simulink model "ft33_project2"  (R2024a)
settings: Solver=VariableStepAuto  StartTime=0.0  StopTime=10.0  RelTol=1e-3
undefined symbols (not defined in the file or in its folder): ft33_project2_copy, Subsystem16, xc7z020clg484
libraries: hdlBasic x111, vmcUtilities x1
(part 1 of 2)
settings Model: Creator=ft33  LastModifiedBy=ft33

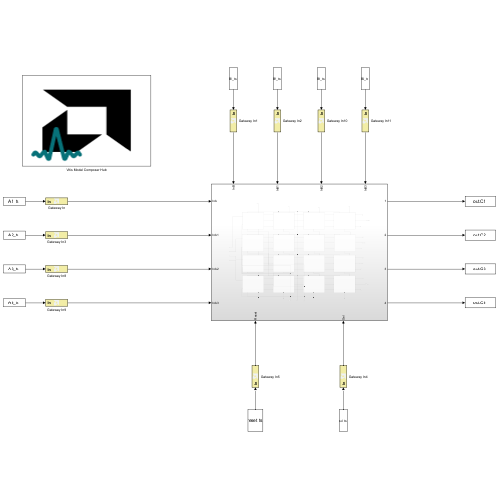
[thumbnail: Simulink's stored preview of the top-level diagram]
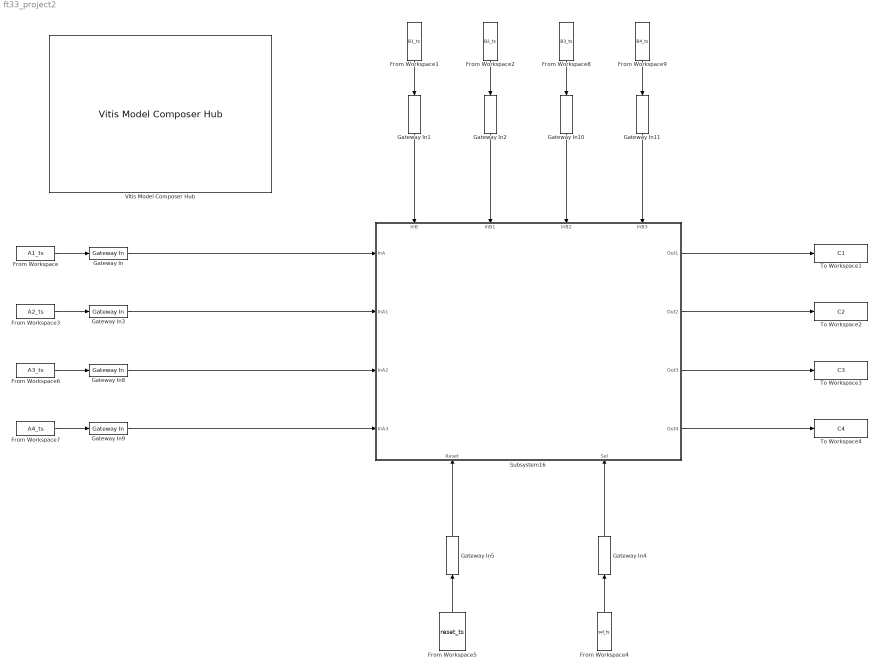
== system ft33_project2 ==
  From Workspace : FromWorkspace  VariableName=A1_ts
  From Workspace1 : FromWorkspace  VariableName=B1_ts
  From Workspace2 : FromWorkspace  VariableName=B2_ts
  From Workspace3 : FromWorkspace  VariableName=A2_ts
  From Workspace4 : FromWorkspace  VariableName=sel_ts
  From Workspace5 : FromWorkspace  VariableName=reset_ts
  From Workspace6 : FromWorkspace  VariableName=A3_ts
  From Workspace7 : FromWorkspace  VariableName=A4_ts
  From Workspace8 : FromWorkspace  VariableName=B3_ts
  From Workspace9 : FromWorkspace  VariableName=B4_ts
  Gateway In{,1..3,8..11} (8 alike) : hdlBasic/Gateway In  gui_display_data_type=Fixed-point  arith_type=Signed (2's comp)  n_bits=16  bin_pt=0  preci_type=Single  exp_width=8  frac_width=24  rows=1  columns=1  quantization="Round  (unbiased: +/- Inf)"  overflow=Saturate  period=1  UseAsADC=off  ADCChannel='1'  interface=None  automatic_assignment=on  address_offset=hex2dec('00')  intf_name=''  intf_description=''  default_value=0  timing_constraint=None  locs_specified=off  LOCs={}  io_standard={}  inherit_from_input=off  hdl_port=on  XmcBlockStatus=1  maskContainerNames=group4  block_type=gatewayin  block_config=sysgen:gateway_in_config  block_width_w=590  block_height_w=620  block_width=640  block_height=850
  Gateway In4 : hdlBasic/Gateway In  gui_display_data_type=Boolean  arith_type=Boolean  n_bits=16  bin_pt=14  preci_type=Single  exp_width=8  frac_width=24  rows=1  columns=1  quantization="Round  (unbiased: +/- Inf)"  overflow=Saturate  period=1  UseAsADC=off  ADCChannel='1'  interface=None  automatic_assignment=on  address_offset=hex2dec('00')  intf_name=''  intf_description=''  default_value=0  timing_constraint=None  locs_specified=off  LOCs={}  io_standard={}  inherit_from_input=off  hdl_port=on  XmcBlockStatus=1  maskContainerNames=group4  block_type=gatewayin  block_config=sysgen:gateway_in_config  block_width_w=590  block_height_w=620  block_width=640  block_height=850
  Gateway In5 : hdlBasic/Gateway In  gui_display_data_type=Boolean  arith_type=Boolean  n_bits=16  bin_pt=14  preci_type=Single  exp_width=8  frac_width=24  rows=1  columns=1  quantization="Round  (unbiased: +/- Inf)"  overflow=Saturate  period=1  UseAsADC=off  ADCChannel='1'  interface=None  automatic_assignment=on  address_offset=hex2dec('00')  intf_name=''  intf_description=''  default_value=0  timing_constraint=None  locs_specified=off  LOCs={}  io_standard={}  inherit_from_input=off  hdl_port=on  XmcBlockStatus=1  maskContainerNames=group4  block_type=gatewayin  block_config=sysgen:gateway_in_config  block_width_w=590  block_height_w=620  block_width=640  block_height=850
  Subsystem16 : Subsystem
      settings: PortSchema="{\"entries\":[{\"content\":{\"sides\":[{\"content\":{\"connectorIds\":[\"In1\",\"In2\",\"In3\",\"In4\"]},\"type\":\"ConnectorPlacement.EquallySpacedRectSide\",\"uuid\":\"57fd51eb-b579-40c5-a499-8811be9ed02c\"},{\"content\":{\"connectorIds\":[\"Out1\",\"Out2\",\"Out3\",\"Out4\"],\"side\":\"RIGHT\"},\"type\":\"ConnectorPlacement.EquallySpacedRectSide\",\"uuid\":\"f81d02a0-f624-4ba0-87e4-de8c38e96c8a\"},{\"content\":{\"connectorIds\":[\"In5\",\"In6\",\"In7\",\"In8\"],\"side\":\"TOP\"},\"type\":\"ConnectorPlacement.EquallySpacedRectSide\",\"uuid\":\"b728b957-3fa5-4fc3-9d0e-7e74a65ebaf5\"},{\"content\":{\"connectorIds\":[\"In9\",\"In10\"],\"side\":\"BOTTOM\"},\"type\":\"ConnectorPlacement.EquallySpacedRectSide\",\"uuid\":\"48c0373e-0401-44d8-8aa7-85e5a3af1fce\"}]},\"type\":\"ConnectorPlacement.EquallySpacedConnector\",\"uuid\":\"375c5da9-2b8b-40e9-8e99-56d50ddf0ba4\"}],\"packageUris\":[\"http://schema.mathworks.com/mf0/Connector/R2020b\"],\"version\":\"1.0\"}"
  To Workspace1 : ToWorkspace  VariableName=C1  SampleTime=-1
  To Workspace2 : ToWorkspace  VariableName=C2  SampleTime=-1
  To Workspace3 : ToWorkspace  VariableName=C3  SampleTime=-1
  To Workspace4 : ToWorkspace  VariableName=C4  SampleTime=-1
  Vitis Model Composer Hub : vmcUtilities/Vitis Model Composer Hub  Tag=genX  CodeGeneration=off  SubsystemName=Subsystem16  BlockHierPath=ft33_project2_copy/Subsystem16  CompilationType=HDLCompilation  SubsystemType=HDLNode  ExportTypeV2=IP Catalog  StartColumn=1  NumberOfColumns=1  TargetDirectory=C:/ELEC522/ft33/Project2_Copy/ResourceAnalysis  exportDesign=off  analyzeDesign=on  validateDesignOnHw=off  ExportType=AI Engines  IpVendor=xilinx.com  IpLibrary=hls  IpVersion=1.0  IpHWLanguage=Verilog  AieCompilerOptions={}  AieSimulatorOptions={}  CreateTestbench=on  TestbenchStackSize=10  RunRtlSim=off  RunCSim=off  RunAieSim=off  AieSimTimeout=50000  RunAieSimProfiling=off  LaunchVitisAnalyzer=off  PlotOutput=off  RunX86Sim=off  X86SimTimeout=10  GenHwImage=off  GenLibadfXo=off  GenHwValidationCode=off  PlatformType=Not Specified  HwSystemType=Baremetal  HwValidationTarget=hw  ProjDevice=ZedBoard Zynq Evaluation and Development Kit (xc7z020clg484-1)  ProjDevicePart=xc7z020clg484-1  AIEType=None  SamplePeriod=-1  ClockFrequency=200  DataPathParallelism=1  xilinxfamily=zynq  part=xc7z020  speed=-1  package=clg484  directory=C:/ELEC522/ft33/Project2_Copy/ResourceAnalysis\ip\Subsystem16\src  testbench=on  incr_netlist=off  synthesis_tool=Vivado  clock_wrapper=Clock Enables  dbl_ovrd=According to Block Masks  dcm_input_clock_period=10  sysclk_period=10  simulink_period=1  eval_field=0  IPInfoJsonString="{\"DUTSubsystemName\":\"Subsystem16\",\"HDLSubsystem\":{\"SubsystemName\":\"Subsystem16\",\"IPName\":\"Subsystem16\",\"IPLibrary\":\"VMC\",\"IPVendor\":\"User Company\",\"IPVersion\":\"1.0\",\"TargetDirectory\":\"C:/ELEC522/ft33/Project2_Copy/ResourceAnalysis\",\"SubsystemDir\":\"C:/ELEC522/ft33/Project2_Copy/ResourceAnalysis\\\\ip\\\\Subsystem16\",\"FreqHz\":\"100000000\"},\"SubsystemTag\":\"HDLNode\"}"  LogFileName=C:\ELEC522\ft33\Project2_Copy\ResourceAnalysis\model_composer.log  NThreads=4  IPConfigFile=C:\Users\ft33\AppData\Local\Temp\vmctmp-8900646231309001291\ft33_project2_copy_ipconfig.json
  wires:
  From Workspace/1 -> Gateway In/1
  From Workspace1/1 -> Gateway In1/1
  From Workspace2/1 -> Gateway In2/1
  From Workspace4/1 -> Gateway In4/1
  From Workspace5/1 -> Gateway In5/1
  From Workspace6/1 -> Gateway In8/1
  From Workspace7/1 -> Gateway In9/1
  From Workspace8/1 -> Gateway In10/1
  From Workspace9/1 -> Gateway In11/1
  From Workspace3/1 -> Gateway In3/1
  Gateway In1/1 -> Subsystem16/5(InB)
  Gateway In2/1 -> Subsystem16/6(InB1)
  Gateway In10/1 -> Subsystem16/7(InB2)
  Gateway In11/1 -> Subsystem16/8(InB3)
  Gateway In/1 -> Subsystem16/1(InA)
  Gateway In3/1 -> Subsystem16/2(InA1)
  Gateway In8/1 -> Subsystem16/3(InA2)
  Gateway In9/1 -> Subsystem16/4(InA3)
  Gateway In4/1 -> Subsystem16/10(Sel)
  Gateway In5/1 -> Subsystem16/9(Reset)
  Subsystem16/1(Out1) -> To Workspace1/1
  Subsystem16/2(Out2) -> To Workspace2/1
  Subsystem16/3(Out3) -> To Workspace3/1
  Subsystem16/4(Out4) -> To Workspace4/1

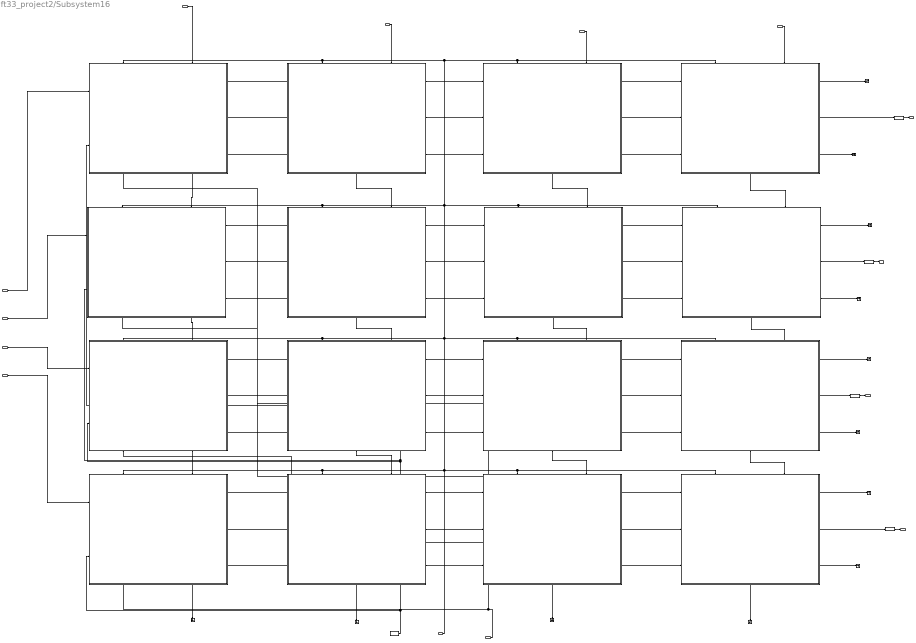
== system ft33_project2/Subsystem16 ==
  InA : Inport
  InA1 : Inport  Port=2
  InA2 : Inport  Port=3
  InA3 : Inport  Port=4
  InB : Inport  Port=5
  InB1 : Inport  Port=6
  InB2 : Inport  Port=7
  InB3 : Inport  Port=8
  Reset : Inport  Port=9
  Sel : Inport  Port=10
  Constant : hdlBasic/Constant  const=0  gui_display_data_type=Fixed-point  arith_type=Unsigned  n_bits=16  bin_pt=0  preci_type=Single  exp_width=8  frac_width=24  explicit_period=off  period=1  XmcBlockStatus=1  maskContainerNames=tabcontainer1  block_type=constant  block_config=sysgen:Constant_config
  Gateway Out{1..4} (4 alike) : hdlBasic/Gateway Out  inherit_from_input=off  bool_to_boolean=off  hdl_port=on  rows=1  columns=1  UseAsDAC=off  DACChannel='1'  interface=None  automatic_assignment=on  address_offset=hex2dec('00')  intf_name=''  intf_description=''  timing_constraint=None  locs_specified=off  LOCs={}  io_standard={}  XmcBlockStatus=1  maskContainerNames=group4  block_type=gatewayout  block_config=sysgen:gateway_out_config  block_width_w=590  block_height_w=620  block_width=620  block_height=750
  Subsystem : Subsystem
      settings: PortSchema="{\"entries\":[{\"content\":{\"sides\":[{\"content\":{\"connectorIds\":[\"In1\",\"In2\"]},\"type\":\"ConnectorPlacement.EquallySpacedRectSide\",\"uuid\":\"273aa0e1-58eb-4403-bf5b-6776102820e6\"},{\"content\":{\"connectorIds\":[\"Out1\",\"Out2\",\"Out3\"],\"side\":\"RIGHT\"},\"type\":\"ConnectorPlacement.EquallySpacedRectSide\",\"uuid\":\"5c33fd88-0c62-4daf-a6d0-9a1459fa340e\"},{\"content\":{\"connectorIds\":[\"In3\",\"In4\"],\"side\":\"TOP\"},\"type\":\"ConnectorPlacement.EquallySpacedRectSide\",\"uuid\":\"2690377b-a45b-49c1-9b26-3eb080cd9126\"},{\"content\":{\"connectorIds\":[\"In5\",\"Out4\"],\"side\":\"BOTTOM\"},\"type\":\"ConnectorPlacement.EquallySpacedRectSide\",\"uuid\":\"fadedb7c-b790-413e-aa9f-7f3073b39ea6\"}]},\"type\":\"ConnectorPlacement.EquallySpacedConnector\",\"uuid\":\"6510aed3-e923-4205-a634-903eef17da44\"}],\"packageUris\":[\"http://schema.mathworks.com/mf0/Connector/R2020b\"],\"version\":\"1.0\"}"
  Subsystem1 : Subsystem
      settings: PortSchema="{\"entries\":[{\"content\":{\"sides\":[{\"content\":{\"connectorIds\":[\"In1\",\"In2\",\"In3\"]},\"type\":\"ConnectorPlacement.EquallySpacedRectSide\",\"uuid\":\"273aa0e1-58eb-4403-bf5b-6776102820e6\"},{\"content\":{\"connectorIds\":[\"Out1\",\"Out2\",\"Out3\"],\"side\":\"RIGHT\"},\"type\":\"ConnectorPlacement.EquallySpacedRectSide\",\"uuid\":\"5c33fd88-0c62-4daf-a6d0-9a1459fa340e\"},{\"content\":{\"connectorIds\":[\"In4\",\"In5\"],\"side\":\"TOP\"},\"type\":\"ConnectorPlacement.EquallySpacedRectSide\",\"uuid\":\"2690377b-a45b-49c1-9b26-3eb080cd9126\"},{\"content\":{\"connectorIds\":[\"Out4\"],\"side\":\"BOTTOM\"},\"type\":\"ConnectorPlacement.EquallySpacedRectSide\",\"uuid\":\"fadedb7c-b790-413e-aa9f-7f3073b39ea6\"}]},\"type\":\"ConnectorPlacement.EquallySpacedConnector\",\"uuid\":\"6510aed3-e923-4205-a634-903eef17da44\"}],\"packageUris\":[\"http://schema.mathworks.com/mf0/Connector/R2020b\"],\"version\":\"1.0\"}"
  Subsystem10 : Subsystem
      settings: PortSchema="{\"entries\":[{\"content\":{\"sides\":[{\"content\":{\"connectorIds\":[\"In1\",\"In2\",\"In3\"]},\"type\":\"ConnectorPlacement.EquallySpacedRectSide\",\"uuid\":\"273aa0e1-58eb-4403-bf5b-6776102820e6\"},{\"content\":{\"connectorIds\":[\"Out1\",\"Out2\",\"Out3\"],\"side\":\"RIGHT\"},\"type\":\"ConnectorPlacement.EquallySpacedRectSide\",\"uuid\":\"5c33fd88-0c62-4daf-a6d0-9a1459fa340e\"},{\"content\":{\"connectorIds\":[\"In4\",\"In5\"],\"side\":\"TOP\"},\"type\":\"ConnectorPlacement.EquallySpacedRectSide\",\"uuid\":\"2690377b-a45b-49c1-9b26-3eb080cd9126\"},{\"content\":{\"connectorIds\":[\"Out4\"],\"side\":\"BOTTOM\"},\"type\":\"ConnectorPlacement.EquallySpacedRectSide\",\"uuid\":\"fadedb7c-b790-413e-aa9f-7f3073b39ea6\"}]},\"type\":\"ConnectorPlacement.EquallySpacedConnector\",\"uuid\":\"6510aed3-e923-4205-a634-903eef17da44\"}],\"packageUris\":[\"http://schema.mathworks.com/mf0/Connector/R2020b\"],\"version\":\"1.0\"}"
  Subsystem11 : Subsystem
      settings: PortSchema="{\"entries\":[{\"content\":{\"sides\":[{\"content\":{\"connectorIds\":[\"In1\",\"In2\",\"In3\"]},\"type\":\"ConnectorPlacement.EquallySpacedRectSide\",\"uuid\":\"273aa0e1-58eb-4403-bf5b-6776102820e6\"},{\"content\":{\"connectorIds\":[\"Out1\",\"Out2\",\"Out3\"],\"side\":\"RIGHT\"},\"type\":\"ConnectorPlacement.EquallySpacedRectSide\",\"uuid\":\"5c33fd88-0c62-4daf-a6d0-9a1459fa340e\"},{\"content\":{\"connectorIds\":[\"In4\",\"In5\"],\"side\":\"TOP\"},\"type\":\"ConnectorPlacement.EquallySpacedRectSide\",\"uuid\":\"2690377b-a45b-49c1-9b26-3eb080cd9126\"},{\"content\":{\"connectorIds\":[\"Out4\"],\"side\":\"BOTTOM\"},\"type\":\"ConnectorPlacement.EquallySpacedRectSide\",\"uuid\":\"fadedb7c-b790-413e-aa9f-7f3073b39ea6\"}]},\"type\":\"ConnectorPlacement.EquallySpacedConnector\",\"uuid\":\"6510aed3-e923-4205-a634-903eef17da44\"}],\"packageUris\":[\"http://schema.mathworks.com/mf0/Connector/R2020b\"],\"version\":\"1.0\"}"
  Subsystem12 : Subsystem
      settings: PortSchema="{\"entries\":[{\"content\":{\"sides\":[{\"content\":{\"connectorIds\":[\"In1\",\"In2\",\"In3\"]},\"type\":\"ConnectorPlacement.EquallySpacedRectSide\",\"uuid\":\"273aa0e1-58eb-4403-bf5b-6776102820e6\"},{\"content\":{\"connectorIds\":[\"Out1\",\"Out2\",\"Out3\"],\"side\":\"RIGHT\"},\"type\":\"ConnectorPlacement.EquallySpacedRectSide\",\"uuid\":\"5c33fd88-0c62-4daf-a6d0-9a1459fa340e\"},{\"content\":{\"connectorIds\":[\"In4\",\"In5\"],\"side\":\"TOP\"},\"type\":\"ConnectorPlacement.EquallySpacedRectSide\",\"uuid\":\"2690377b-a45b-49c1-9b26-3eb080cd9126\"},{\"content\":{\"connectorIds\":[\"Out4\"],\"side\":\"BOTTOM\"},\"type\":\"ConnectorPlacement.EquallySpacedRectSide\",\"uuid\":\"fadedb7c-b790-413e-aa9f-7f3073b39ea6\"}]},\"type\":\"ConnectorPlacement.EquallySpacedConnector\",\"uuid\":\"6510aed3-e923-4205-a634-903eef17da44\"}],\"packageUris\":[\"http://schema.mathworks.com/mf0/Connector/R2020b\"],\"version\":\"1.0\"}"
  Subsystem13 : Subsystem
      settings: PortSchema="{\"entries\":[{\"content\":{\"sides\":[{\"content\":{\"connectorIds\":[\"In1\",\"In2\",\"In3\"]},\"type\":\"ConnectorPlacement.EquallySpacedRectSide\",\"uuid\":\"273aa0e1-58eb-4403-bf5b-6776102820e6\"},{\"content\":{\"connectorIds\":[\"Out1\",\"Out2\",\"Out3\"],\"side\":\"RIGHT\"},\"type\":\"ConnectorPlacement.EquallySpacedRectSide\",\"uuid\":\"5c33fd88-0c62-4daf-a6d0-9a1459fa340e\"},{\"content\":{\"connectorIds\":[\"In4\",\"In5\"],\"side\":\"TOP\"},\"type\":\"ConnectorPlacement.EquallySpacedRectSide\",\"uuid\":\"2690377b-a45b-49c1-9b26-3eb080cd9126\"},{\"content\":{\"connectorIds\":[\"Out4\"],\"side\":\"BOTTOM\"},\"type\":\"ConnectorPlacement.EquallySpacedRectSide\",\"uuid\":\"fadedb7c-b790-413e-aa9f-7f3073b39ea6\"}]},\"type\":\"ConnectorPlacement.EquallySpacedConnector\",\"uuid\":\"6510aed3-e923-4205-a634-903eef17da44\"}],\"packageUris\":[\"http://schema.mathworks.com/mf0/Connector/R2020b\"],\"version\":\"1.0\"}"
  Subsystem14 : Subsystem
      settings: PortSchema="{\"entries\":[{\"content\":{\"sides\":[{\"content\":{\"connectorIds\":[\"In1\",\"In2\",\"In3\"]},\"type\":\"ConnectorPlacement.EquallySpacedRectSide\",\"uuid\":\"273aa0e1-58eb-4403-bf5b-6776102820e6\"},{\"content\":{\"connectorIds\":[\"Out1\",\"Out2\",\"Out3\"],\"side\":\"RIGHT\"},\"type\":\"ConnectorPlacement.EquallySpacedRectSide\",\"uuid\":\"5c33fd88-0c62-4daf-a6d0-9a1459fa340e\"},{\"content\":{\"connectorIds\":[\"In4\",\"In5\"],\"side\":\"TOP\"},\"type\":\"ConnectorPlacement.EquallySpacedRectSide\",\"uuid\":\"2690377b-a45b-49c1-9b26-3eb080cd9126\"},{\"content\":{\"connectorIds\":[\"Out4\"],\"side\":\"BOTTOM\"},\"type\":\"ConnectorPlacement.EquallySpacedRectSide\",\"uuid\":\"fadedb7c-b790-413e-aa9f-7f3073b39ea6\"}]},\"type\":\"ConnectorPlacement.EquallySpacedConnector\",\"uuid\":\"6510aed3-e923-4205-a634-903eef17da44\"}],\"packageUris\":[\"http://schema.mathworks.com/mf0/Connector/R2020b\"],\"version\":\"1.0\"}"
  Subsystem15 : Subsystem
      settings: PortSchema="{\"entries\":[{\"content\":{\"sides\":[{\"content\":{\"connectorIds\":[\"In1\",\"In2\",\"In3\"]},\"type\":\"ConnectorPlacement.EquallySpacedRectSide\",\"uuid\":\"273aa0e1-58eb-4403-bf5b-6776102820e6\"},{\"content\":{\"connectorIds\":[\"Out1\",\"Out2\",\"Out3\"],\"side\":\"RIGHT\"},\"type\":\"ConnectorPlacement.EquallySpacedRectSide\",\"uuid\":\"5c33fd88-0c62-4daf-a6d0-9a1459fa340e\"},{\"content\":{\"connectorIds\":[\"In4\",\"In5\"],\"side\":\"TOP\"},\"type\":\"ConnectorPlacement.EquallySpacedRectSide\",\"uuid\":\"2690377b-a45b-49c1-9b26-3eb080cd9126\"},{\"content\":{\"connectorIds\":[\"Out4\"],\"side\":\"BOTTOM\"},\"type\":\"ConnectorPlacement.EquallySpacedRectSide\",\"uuid\":\"fadedb7c-b790-413e-aa9f-7f3073b39ea6\"}]},\"type\":\"ConnectorPlacement.EquallySpacedConnector\",\"uuid\":\"6510aed3-e923-4205-a634-903eef17da44\"}],\"packageUris\":[\"http://schema.mathworks.com/mf0/Connector/R2020b\"],\"version\":\"1.0\"}"
  Subsystem2 : Subsystem
      settings: PortSchema="{\"entries\":[{\"content\":{\"sides\":[{\"content\":{\"connectorIds\":[\"In1\",\"In2\"]},\"type\":\"ConnectorPlacement.EquallySpacedRectSide\",\"uuid\":\"273aa0e1-58eb-4403-bf5b-6776102820e6\"},{\"content\":{\"connectorIds\":[\"Out1\",\"Out2\",\"Out3\"],\"side\":\"RIGHT\"},\"type\":\"ConnectorPlacement.EquallySpacedRectSide\",\"uuid\":\"5c33fd88-0c62-4daf-a6d0-9a1459fa340e\"},{\"content\":{\"connectorIds\":[\"In3\",\"In4\"],\"side\":\"TOP\"},\"type\":\"ConnectorPlacement.EquallySpacedRectSide\",\"uuid\":\"2690377b-a45b-49c1-9b26-3eb080cd9126\"},{\"content\":{\"connectorIds\":[\"In5\",\"Out4\"],\"side\":\"BOTTOM\"},\"type\":\"ConnectorPlacement.EquallySpacedRectSide\",\"uuid\":\"fadedb7c-b790-413e-aa9f-7f3073b39ea6\"}]},\"type\":\"ConnectorPlacement.EquallySpacedConnector\",\"uuid\":\"6510aed3-e923-4205-a634-903eef17da44\"}],\"packageUris\":[\"http://schema.mathworks.com/mf0/Connector/R2020b\"],\"version\":\"1.0\"}"
  Subsystem3 : Subsystem
      settings: PortSchema="{\"entries\":[{\"content\":{\"sides\":[{\"content\":{\"connectorIds\":[\"In1\",\"In2\",\"In3\"]},\"type\":\"ConnectorPlacement.EquallySpacedRectSide\",\"uuid\":\"273aa0e1-58eb-4403-bf5b-6776102820e6\"},{\"content\":{\"connectorIds\":[\"Out1\",\"Out2\",\"Out3\"],\"side\":\"RIGHT\"},\"type\":\"ConnectorPlacement.EquallySpacedRectSide\",\"uuid\":\"5c33fd88-0c62-4daf-a6d0-9a1459fa340e\"},{\"content\":{\"connectorIds\":[\"In4\",\"In5\"],\"side\":\"TOP\"},\"type\":\"ConnectorPlacement.EquallySpacedRectSide\",\"uuid\":\"2690377b-a45b-49c1-9b26-3eb080cd9126\"},{\"content\":{\"connectorIds\":[\"Out4\"],\"side\":\"BOTTOM\"},\"type\":\"ConnectorPlacement.EquallySpacedRectSide\",\"uuid\":\"fadedb7c-b790-413e-aa9f-7f3073b39ea6\"}]},\"type\":\"ConnectorPlacement.EquallySpacedConnector\",\"uuid\":\"6510aed3-e923-4205-a634-903eef17da44\"}],\"packageUris\":[\"http://schema.mathworks.com/mf0/Connector/R2020b\"],\"version\":\"1.0\"}"
  Subsystem4 : Subsystem
      settings: PortSchema="{\"entries\":[{\"content\":{\"sides\":[{\"content\":{\"connectorIds\":[\"In1\",\"In2\"]},\"type\":\"ConnectorPlacement.EquallySpacedRectSide\",\"uuid\":\"273aa0e1-58eb-4403-bf5b-6776102820e6\"},{\"content\":{\"connectorIds\":[\"Out1\",\"Out2\",\"Out3\"],\"side\":\"RIGHT\"},\"type\":\"ConnectorPlacement.EquallySpacedRectSide\",\"uuid\":\"5c33fd88-0c62-4daf-a6d0-9a1459fa340e\"},{\"content\":{\"connectorIds\":[\"In3\",\"In4\"],\"side\":\"TOP\"},\"type\":\"ConnectorPlacement.EquallySpacedRectSide\",\"uuid\":\"2690377b-a45b-49c1-9b26-3eb080cd9126\"},{\"content\":{\"connectorIds\":[\"In5\",\"Out4\"],\"side\":\"BOTTOM\"},\"type\":\"ConnectorPlacement.EquallySpacedRectSide\",\"uuid\":\"fadedb7c-b790-413e-aa9f-7f3073b39ea6\"}]},\"type\":\"ConnectorPlacement.EquallySpacedConnector\",\"uuid\":\"6510aed3-e923-4205-a634-903eef17da44\"}],\"packageUris\":[\"http://schema.mathworks.com/mf0/Connector/R2020b\"],\"version\":\"1.0\"}"
  Subsystem5 : Subsystem
      settings: PortSchema="{\"entries\":[{\"content\":{\"sides\":[{\"content\":{\"connectorIds\":[\"In1\",\"In2\"]},\"type\":\"ConnectorPlacement.EquallySpacedRectSide\",\"uuid\":\"273aa0e1-58eb-4403-bf5b-6776102820e6\"},{\"content\":{\"connectorIds\":[\"Out1\",\"Out2\",\"Out3\"],\"side\":\"RIGHT\"},\"type\":\"ConnectorPlacement.EquallySpacedRectSide\",\"uuid\":\"5c33fd88-0c62-4daf-a6d0-9a1459fa340e\"},{\"content\":{\"connectorIds\":[\"In3\",\"In4\"],\"side\":\"TOP\"},\"type\":\"ConnectorPlacement.EquallySpacedRectSide\",\"uuid\":\"2690377b-a45b-49c1-9b26-3eb080cd9126\"},{\"content\":{\"connectorIds\":[\"In5\",\"Out4\"],\"side\":\"BOTTOM\"},\"type\":\"ConnectorPlacement.EquallySpacedRectSide\",\"uuid\":\"fadedb7c-b790-413e-aa9f-7f3073b39ea6\"}]},\"type\":\"ConnectorPlacement.EquallySpacedConnector\",\"uuid\":\"6510aed3-e923-4205-a634-903eef17da44\"}],\"packageUris\":[\"http://schema.mathworks.com/mf0/Connector/R2020b\"],\"version\":\"1.0\"}"
  Subsystem6 : Subsystem
      settings: PortSchema="{\"entries\":[{\"content\":{\"sides\":[{\"content\":{\"connectorIds\":[\"In1\",\"In2\",\"In3\"]},\"type\":\"ConnectorPlacement.EquallySpacedRectSide\",\"uuid\":\"273aa0e1-58eb-4403-bf5b-6776102820e6\"},{\"content\":{\"connectorIds\":[\"Out1\",\"Out2\",\"Out3\"],\"side\":\"RIGHT\"},\"type\":\"ConnectorPlacement.EquallySpacedRectSide\",\"uuid\":\"5c33fd88-0c62-4daf-a6d0-9a1459fa340e\"},{\"content\":{\"connectorIds\":[\"In4\",\"In5\"],\"side\":\"TOP\"},\"type\":\"ConnectorPlacement.EquallySpacedRectSide\",\"uuid\":\"2690377b-a45b-49c1-9b26-3eb080cd9126\"},{\"content\":{\"connectorIds\":[\"Out4\"],\"side\":\"BOTTOM\"},\"type\":\"ConnectorPlacement.EquallySpacedRectSide\",\"uuid\":\"fadedb7c-b790-413e-aa9f-7f3073b39ea6\"}]},\"type\":\"ConnectorPlacement.EquallySpacedConnector\",\"uuid\":\"6510aed3-e923-4205-a634-903eef17da44\"}],\"packageUris\":[\"http://schema.mathworks.com/mf0/Connector/R2020b\"],\"version\":\"1.0\"}"
  Subsystem7 : Subsystem
      settings: PortSchema="{\"entries\":[{\"content\":{\"sides\":[{\"content\":{\"connectorIds\":[\"In1\",\"In2\",\"In3\"]},\"type\":\"ConnectorPlacement.EquallySpacedRectSide\",\"uuid\":\"273aa0e1-58eb-4403-bf5b-6776102820e6\"},{\"content\":{\"connectorIds\":[\"Out1\",\"Out2\",\"Out3\"],\"side\":\"RIGHT\"},\"type\":\"ConnectorPlacement.EquallySpacedRectSide\",\"uuid\":\"5c33fd88-0c62-4daf-a6d0-9a1459fa340e\"},{\"content\":{\"connectorIds\":[\"In4\",\"In5\"],\"side\":\"TOP\"},\"type\":\"ConnectorPlacement.EquallySpacedRectSide\",\"uuid\":\"2690377b-a45b-49c1-9b26-3eb080cd9126\"},{\"content\":{\"connectorIds\":[\"Out4\"],\"side\":\"BOTTOM\"},\"type\":\"ConnectorPlacement.EquallySpacedRectSide\",\"uuid\":\"fadedb7c-b790-413e-aa9f-7f3073b39ea6\"}]},\"type\":\"ConnectorPlacement.EquallySpacedConnector\",\"uuid\":\"6510aed3-e923-4205-a634-903eef17da44\"}],\"packageUris\":[\"http://schema.mathworks.com/mf0/Connector/R2020b\"],\"version\":\"1.0\"}"
  Subsystem8 : Subsystem
      settings: PortSchema="{\"entries\":[{\"content\":{\"sides\":[{\"content\":{\"connectorIds\":[\"In1\",\"In2\",\"In3\"]},\"type\":\"ConnectorPlacement.EquallySpacedRectSide\",\"uuid\":\"273aa0e1-58eb-4403-bf5b-6776102820e6\"},{\"content\":{\"connectorIds\":[\"Out1\",\"Out2\",\"Out3\"],\"side\":\"RIGHT\"},\"type\":\"ConnectorPlacement.EquallySpacedRectSide\",\"uuid\":\"5c33fd88-0c62-4daf-a6d0-9a1459fa340e\"},{\"content\":{\"connectorIds\":[\"In4\",\"In5\"],\"side\":\"TOP\"},\"type\":\"ConnectorPlacement.EquallySpacedRectSide\",\"uuid\":\"2690377b-a45b-49c1-9b26-3eb080cd9126\"},{\"content\":{\"connectorIds\":[\"Out4\"],\"side\":\"BOTTOM\"},\"type\":\"ConnectorPlacement.EquallySpacedRectSide\",\"uuid\":\"fadedb7c-b790-413e-aa9f-7f3073b39ea6\"}]},\"type\":\"ConnectorPlacement.EquallySpacedConnector\",\"uuid\":\"6510aed3-e923-4205-a634-903eef17da44\"}],\"packageUris\":[\"http://schema.mathworks.com/mf0/Connector/R2020b\"],\"version\":\"1.0\"}"
  Subsystem9 : Subsystem
      settings: PortSchema="{\"entries\":[{\"content\":{\"sides\":[{\"content\":{\"connectorIds\":[\"In1\",\"In2\",\"In3\"]},\"type\":\"ConnectorPlacement.EquallySpacedRectSide\",\"uuid\":\"273aa0e1-58eb-4403-bf5b-6776102820e6\"},{\"content\":{\"connectorIds\":[\"Out1\",\"Out2\",\"Out3\"],\"side\":\"RIGHT\"},\"type\":\"ConnectorPlacement.EquallySpacedRectSide\",\"uuid\":\"5c33fd88-0c62-4daf-a6d0-9a1459fa340e\"},{\"content\":{\"connectorIds\":[\"In4\",\"In5\"],\"side\":\"TOP\"},\"type\":\"ConnectorPlacement.EquallySpacedRectSide\",\"uuid\":\"2690377b-a45b-49c1-9b26-3eb080cd9126\"},{\"content\":{\"connectorIds\":[\"Out4\"],\"side\":\"BOTTOM\"},\"type\":\"ConnectorPlacement.EquallySpacedRectSide\",\"uuid\":\"fadedb7c-b790-413e-aa9f-7f3073b39ea6\"}]},\"type\":\"ConnectorPlacement.EquallySpacedConnector\",\"uuid\":\"6510aed3-e923-4205-a634-903eef17da44\"}],\"packageUris\":[\"http://schema.mathworks.com/mf0/Connector/R2020b\"],\"version\":\"1.0\"}"
  Terminator{,1..11} (12 alike) : Terminator
  Out1 : Outport
  Out2 : Outport  Port=2
  Out3 : Outport  Port=3
  Out4 : Outport  Port=4
  wires:
  Subsystem5/4(OutB) -> Terminator/1  "ShiftB"
  Reset/1 -> Subsystem5/5(Reset), Subsystem4/5(Reset), Subsystem2/5(Reset), Subsystem/5(ResetIn)
  Subsystem3/1(OutA) -> Subsystem15/1(InA)  "ShiftB"
  Constant/1 -> Subsystem5/2(ShiftIn), Subsystem4/2(ShiftIn), Subsystem2/2(ShiftIn), Subsystem/2(ShiftIn)
  InB2/1 -> Subsystem14/5(InB)
  Subsystem1/1(OutA) -> Subsystem14/1(InA)  "ShiftB"
  Subsystem12/4(OutB) -> Subsystem13/5(InB)  "ShiftB"
  Subsystem6/4(OutB) -> Subsystem7/5(InB)  "ShiftB"
  InB/1 -> Subsystem/4(InB)
  Subsystem13/2(ShiftOut) -> Gateway Out3/1
  Sel/1 -> Subsystem11/4(Select), Subsystem9/4(Select), Subsystem7/4(Select), Subsystem5/3(Select), Subsystem10/4(Select), Subsystem8/4(Select), Subsystem6/4(Select), Subsystem4/3(Select), Subsystem13/4(Select), Subsystem15/4(Select), Subsystem3/4(Select), Subsystem2/3(Select), Subsystem14/4(Select), Subsystem12/4(Select), Subsystem1/4(Select), Subsystem/3(Select)
  Subsystem15/2(ShiftOut) -> Subsystem13/2(ShiftIn)  "ShiftOutput"
  Subsystem13/1(OutA) -> Terminator6/1  "ShiftA"
  InA2/1 -> Subsystem4/1(InA)
  Subsystem11/1(OutA) -> Terminator4/1  "ShiftA"
  Subsystem10/1(OutA) -> Terminator5/1  "ShiftA"
  Subsystem11/4(OutB) -> Terminator3/1  "ShiftB"
  Subsystem14/1(OutA) -> Subsystem12/1(InA)  "ShiftA"
  Subsystem14/4(OutB) -> Subsystem15/5(InB)  "ShiftB"
  Subsystem15/1(OutA) -> Subsystem13/1(InA)  "ShiftA"
  Subsystem3/4(OutB) -> Subsystem6/5(InB)  "ShiftB"
  Subsystem10/2(ShiftOut) -> Gateway Out2/1
  Subsystem7/4(OutB) -> Terminator1/1  "ShiftB"
  Subsystem2/4(OutB) -> Subsystem4/4(InB)  "ShiftB"
  Gateway Out4/1 -> Out4/1
  Subsystem/4(OutB) -> Subsystem2/4(InB)  "ShiftB"
  Subsystem3/2(ShiftOut) -> Subsystem15/2(ShiftIn)  "ShiftA"
  Subsystem/2(ShiftOut) -> Subsystem1/2(ShiftIn)  "ShiftOutput"
  InA/1 -> Subsystem/1(InA)
  Subsystem12/1(OutA) -> Terminator7/1  "ShiftA"
  Subsystem2/2(ShiftOut) -> Subsystem3/2(ShiftIn)  "ShiftOutput"
  Subsystem4/4(OutB) -> Subsystem5/4(InB)  "ShiftB"
  Subsystem8/4(OutB) -> Subsystem9/5(InB)  "ShiftB"
  Subsystem15/4(OutB) -> Subsystem8/5(InB)  "ShiftB"
  Subsystem9/4(OutB) -> Terminator2/1  "ShiftB"
  Subsystem10/4(OutB) -> Subsystem11/5(InB)  "ShiftB"
  Subsystem13/4(OutB) -> Subsystem10/5(InB)  "ShiftB"
  Subsystem1/4(OutB) -> Subsystem3/5(InB)  "ShiftB"
  Subsystem2/1(OutA) -> Subsystem3/1(InA)  "ShiftA"
  InA3/1 -> Subsystem5/1(InA)
  Subsystem/1(OutA) -> Subsystem1/1(InA)  "ShiftA"
  Gateway Out2/1 -> Out3/1
  Gateway Out3/1 -> Out2/1
  Gateway Out1/1 -> Out1/1
  InA1/1 -> Subsystem2/1(InA)
  InB3/1 -> Subsystem12/5(InB)
  InB1/1 -> Subsystem1/5(InB)
  Subsystem1/2(ShiftOut) -> Subsystem14/2(ShiftIn)  "ShiftOutput"
  Subsystem14/2(ShiftOut) -> Subsystem12/2(ShiftIn)  "ShiftOutput"
  Subsystem12/2(ShiftOut) -> Gateway Out1/1  "ShiftOutput"
  Subsystem11/2(ShiftOut) -> Gateway Out4/1  "ShiftOutput"
  Subsystem/3(ResetOut) -> Subsystem1/3(ResetIn)
  Subsystem1/3(Out1) -> Subsystem14/3(ResetIn)
  Subsystem14/3(ResetOut) -> Subsystem12/3(ResetIn)
  Subsystem12/3(ResetOut) -> Terminator8/1
  Subsystem2/3(ResetOut) -> Subsystem3/3(ResetIn)
  Subsystem3/3(ResetOut) -> Subsystem15/3(ResetIn)
  Subsystem15/3(ResetOut) -> Subsystem13/3(ResetIn)
  Subsystem13/3(ResetOut) -> Terminator9/1
  Subsystem4/1(OutA) -> Subsystem6/1(InA)  "ShiftA"
  Subsystem4/2(ShiftOut) -> Subsystem6/2(ShiftIn)  "ShiftOutput"
  Subsystem4/3(ResetOut) -> Subsystem6/3(ResetIn)
  Subsystem6/3(ResetOut) -> Subsystem8/3(ResetIn)
  Subsystem6/2(ShiftOut) -> Subsystem8/2(ShiftIn)  "ShiftA"
  Subsystem6/1(OutA) -> Subsystem8/1(InA)  "ShiftB"
  Subsystem8/1(OutA) -> Subsystem10/1(InA)  "ShiftB"
  Subsystem8/2(ShiftOut) -> Subsystem10/2(ShiftIn)  "ShiftA"
  Subsystem8/3(ResetOut) -> Subsystem10/3(ResetIn)
  Subsystem10/3(ResetOut) -> Terminator10/1
  Subsystem5/1(OutA) -> Subsystem7/1(InA)  "ShiftA"
  Subsystem5/2(ShiftOut) -> Subsystem7/2(ShiftIn)  "ShiftOutput"
  Subsystem5/3(ResetOut) -> Subsystem7/3(ResetIn)
  Subsystem7/1(OutA) -> Subsystem9/1(InA)  "ShiftB"
  Subsystem7/2(ShiftOut) -> Subsystem9/2(ShiftIn)  "ShiftA"
  Subsystem7/3(ResetOut) -> Subsystem9/3(ResetIn)
  Subsystem9/1(OutA) -> Subsystem11/1(InA)  "ShiftB"
  Subsystem9/2(ShiftOut) -> Subsystem11/2(ShiftIn)  "ShiftA"
  Subsystem9/3(ResetOut) -> Subsystem11/3(ResetIn)
  Subsystem11/3(ResetOut) -> Terminator11/1

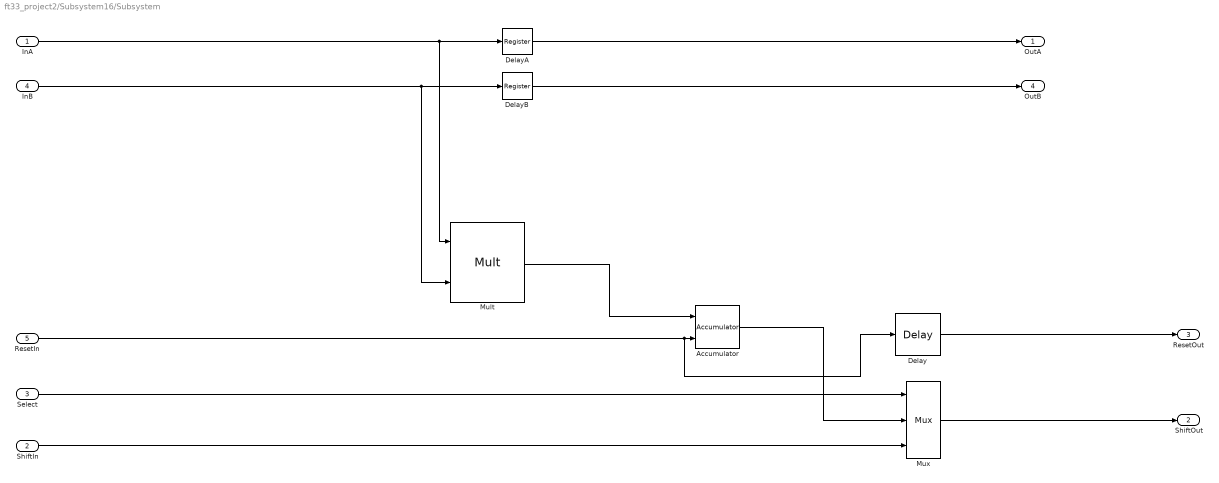
== system ft33_project2/Subsystem16/Subsystem ==
  InA : Inport
  ShiftIn : Inport  Port=2
  Select : Inport  Port=3
  InB : Inport  Port=4
  ResetIn : Inport  Port=5
  Accumulator : hdlBasic/Accumulator  operation=Add  n_bits=16  overflow=Flag as error  scale=1  rst=on  hasbypass=off  en=off  latency=1  msb_inp=100  msb=100  lsb=-100  use_behavioral_HDL=on  implementation=Fabric  XmcBlockStatus=1  maskContainerNames=group3  block_type=accum  block_config=sysgen:Accum_config  block_width=566  block_height=845
  Delay : hdlBasic/Delay  rst=off  en=off  latency=1  reg_retiming=off  XmcBlockStatus=1  maskContainerNames=group1  block_type=delay  block_config=sysgen:Delay_config
  DelayA : hdlBasic/Register  init=0  rst=off  en=off  XmcBlockStatus=1  maskContainerNames=tabcontainer1  block_type=register  block_config=sysgen:Register_config
  DelayB : hdlBasic/Register  init=0  rst=off  en=off  XmcBlockStatus=1  maskContainerNames=tabcontainer1  block_type=register  block_config=sysgen:Register_config
  Mult : hdlBasic/Mult  precision=User Defined  arith_type="Signed  (2's comp)"  n_bits=16  bin_pt=0  quantization=Truncate  overflow=Wrap  en=off  latency=1  opt_float=off  fp_mult_usage=No Usage  use_behavioral_HDL=off  opt=Speed  use_embedded=on  optimum_pipeline=off  pipeline=on  use_rpm=on  placement_style=Triangular  XmcBlockStatus=1  maskContainerNames=group1  block_type=mult  block_config=sysgen:Mult_config  block_width=598  block_height=876
  Mux : hdlBasic/Mux  inputs=2  en=off  latency=1  precision=Full  arith_type=Unsigned  n_bits=16  bin_pt=14  quantization=Truncate  overflow=Wrap  XmcBlockStatus=1  maskContainerNames=tabcontainer1  block_type=mux  block_config=sysgen:Mux_config
  OutA : Outport
  ShiftOut : Outport  Port=2
  ResetOut : Outport  Port=3
  OutB : Outport  Port=4
  wires:
  Accumulator/1 -> Mux/2
  Mult/1 -> Accumulator/1
  InB/1 -> DelayB/1, Mult/2
  Select/1 -> Mux/1
  ShiftIn/1 -> Mux/3
  Mux/1 -> ShiftOut/1
  ResetIn/1 -> Delay/1, Accumulator/2
  InA/1 -> Mult/1, DelayA/1
  DelayA/1 -> OutA/1
  DelayB/1 -> OutB/1
  Delay/1 -> ResetOut/1

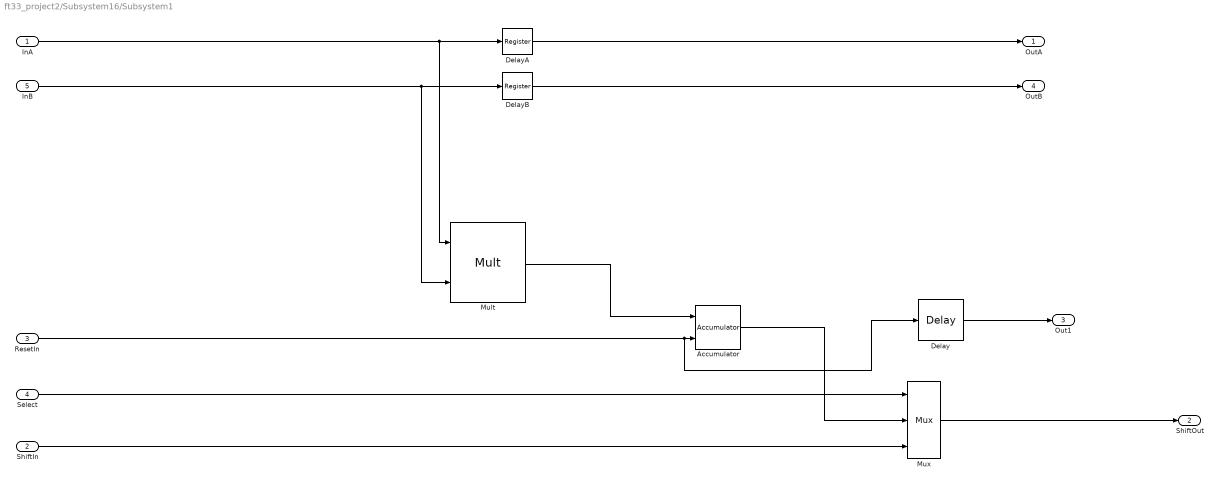
== system ft33_project2/Subsystem16/Subsystem1 ==
  InA : Inport
  ShiftIn : Inport  Port=2
  ResetIn : Inport  Port=3
  Select : Inport  Port=4
  InB : Inport  Port=5
  Accumulator : hdlBasic/Accumulator  operation=Add  n_bits=16  overflow=Wrap  scale=1  rst=on  hasbypass=off  en=off  latency=1  msb_inp=100  msb=100  lsb=-100  use_behavioral_HDL=on  implementation=Fabric  XmcBlockStatus=1  maskContainerNames=group3  block_type=accum  block_config=sysgen:Accum_config  block_width=566  block_height=845
  Delay : hdlBasic/Delay  rst=off  en=off  latency=1  reg_retiming=off  XmcBlockStatus=1  maskContainerNames=group1  block_type=delay  block_config=sysgen:Delay_config
  DelayA : hdlBasic/Register  init=0  rst=off  en=off  XmcBlockStatus=1  maskContainerNames=tabcontainer1  block_type=register  block_config=sysgen:Register_config
  DelayB : hdlBasic/Register  init=0  rst=off  en=off  XmcBlockStatus=1  maskContainerNames=tabcontainer1  block_type=register  block_config=sysgen:Register_config
  Mult : hdlBasic/Mult  precision=User Defined  arith_type="Signed  (2's comp)"  n_bits=16  bin_pt=0  quantization=Truncate  overflow=Wrap  en=off  latency=1  opt_float=off  fp_mult_usage=No Usage  use_behavioral_HDL=off  opt=Speed  use_embedded=on  optimum_pipeline=off  pipeline=on  use_rpm=on  placement_style=Triangular  XmcBlockStatus=1  maskContainerNames=group1  block_type=mult  block_config=sysgen:Mult_config  block_width=598  block_height=876
  Mux : hdlBasic/Mux  inputs=2  en=off  latency=1  precision=Full  arith_type=Unsigned  n_bits=16  bin_pt=14  quantization=Truncate  overflow=Wrap  XmcBlockStatus=1  maskContainerNames=tabcontainer1  block_type=mux  block_config=sysgen:Mux_config
  OutA : Outport
  ShiftOut : Outport  Port=2
  Out1 : Outport  Port=3
  OutB : Outport  Port=4
  wires:
  Accumulator/1 -> Mux/2
  Mult/1 -> Accumulator/1
  InB/1 -> DelayB/1, Mult/2
  Select/1 -> Mux/1
  ShiftIn/1 -> Mux/3
  Mux/1 -> ShiftOut/1
  ResetIn/1 -> Delay/1, Accumulator/2
  InA/1 -> Mult/1, DelayA/1
  DelayA/1 -> OutA/1
  DelayB/1 -> OutB/1
  Delay/1 -> Out1/1

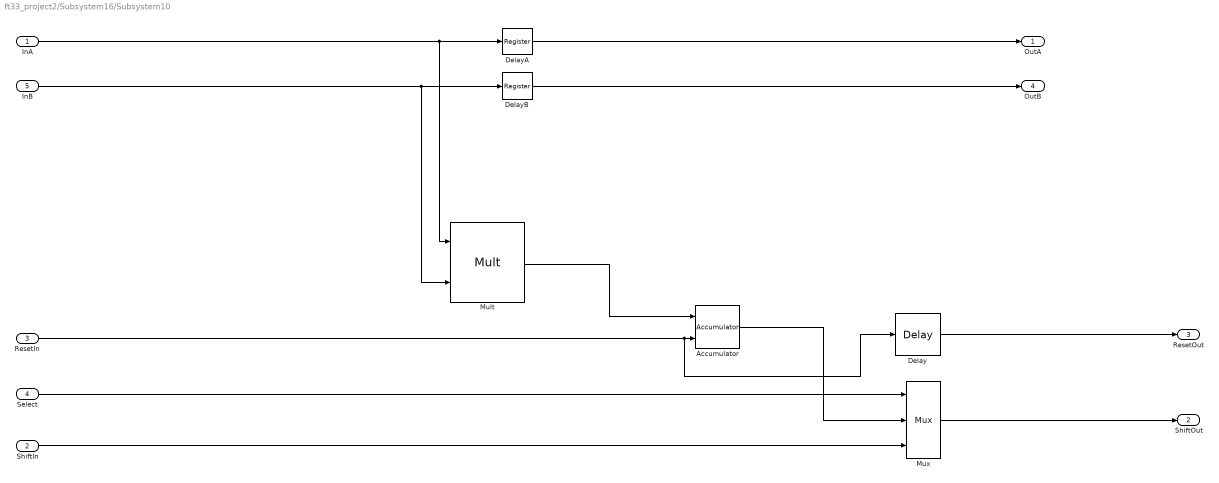
== system ft33_project2/Subsystem16/Subsystem10 ==
  InA : Inport
  ShiftIn : Inport  Port=2
  ResetIn : Inport  Port=3
  Select : Inport  Port=4
  InB : Inport  Port=5
  Accumulator : hdlBasic/Accumulator  operation=Add  n_bits=16  overflow=Flag as error  scale=1  rst=on  hasbypass=off  en=off  latency=1  msb_inp=100  msb=100  lsb=-100  use_behavioral_HDL=on  implementation=Fabric  XmcBlockStatus=1  maskContainerNames=group3  block_type=accum  block_config=sysgen:Accum_config  block_width=566  block_height=845
  Delay : hdlBasic/Delay  rst=off  en=off  latency=1  reg_retiming=off  XmcBlockStatus=1  maskContainerNames=group1  block_type=delay  block_config=sysgen:Delay_config
  DelayA : hdlBasic/Register  init=0  rst=off  en=off  XmcBlockStatus=1  maskContainerNames=tabcontainer1  block_type=register  block_config=sysgen:Register_config
  DelayB : hdlBasic/Register  init=0  rst=off  en=off  XmcBlockStatus=1  maskContainerNames=tabcontainer1  block_type=register  block_config=sysgen:Register_config
  Mult : hdlBasic/Mult  precision=User Defined  arith_type="Signed  (2's comp)"  n_bits=16  bin_pt=0  quantization=Truncate  overflow=Wrap  en=off  latency=1  opt_float=off  fp_mult_usage=No Usage  use_behavioral_HDL=off  opt=Speed  use_embedded=on  optimum_pipeline=off  pipeline=on  use_rpm=on  placement_style=Triangular  XmcBlockStatus=1  maskContainerNames=group1  block_type=mult  block_config=sysgen:Mult_config  block_width=598  block_height=876
  Mux : hdlBasic/Mux  inputs=2  en=off  latency=1  precision=Full  arith_type=Unsigned  n_bits=16  bin_pt=14  quantization=Truncate  overflow=Wrap  XmcBlockStatus=1  maskContainerNames=tabcontainer1  block_type=mux  block_config=sysgen:Mux_config
  OutA : Outport
  ShiftOut : Outport  Port=2
  ResetOut : Outport  Port=3
  OutB : Outport  Port=4
  wires:
  Accumulator/1 -> Mux/2
  Mult/1 -> Accumulator/1
  InB/1 -> DelayB/1, Mult/2
  Select/1 -> Mux/1
  ShiftIn/1 -> Mux/3
  Mux/1 -> ShiftOut/1
  ResetIn/1 -> Delay/1, Accumulator/2
  InA/1 -> Mult/1, DelayA/1
  DelayA/1 -> OutA/1
  DelayB/1 -> OutB/1
  Delay/1 -> ResetOut/1

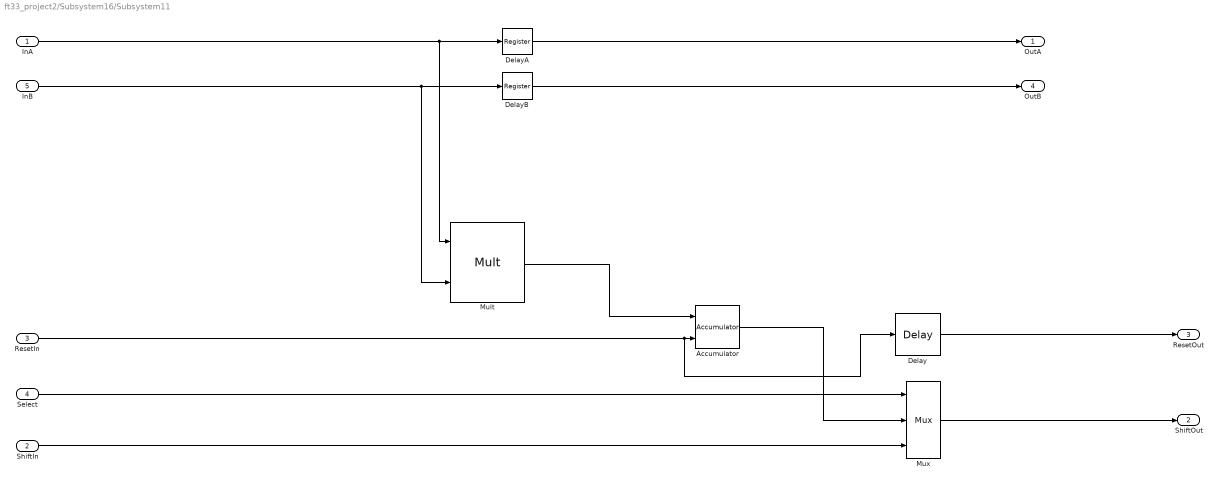
== system ft33_project2/Subsystem16/Subsystem11 ==
  InA : Inport
  ShiftIn : Inport  Port=2
  ResetIn : Inport  Port=3
  Select : Inport  Port=4
  InB : Inport  Port=5
  Accumulator : hdlBasic/Accumulator  operation=Add  n_bits=16  overflow=Flag as error  scale=1  rst=on  hasbypass=off  en=off  latency=1  msb_inp=100  msb=100  lsb=-100  use_behavioral_HDL=on  implementation=Fabric  XmcBlockStatus=1  maskContainerNames=group3  block_type=accum  block_config=sysgen:Accum_config  block_width=566  block_height=845
  Delay : hdlBasic/Delay  rst=off  en=off  latency=1  reg_retiming=off  XmcBlockStatus=1  maskContainerNames=group1  block_type=delay  block_config=sysgen:Delay_config
  DelayA : hdlBasic/Register  init=0  rst=off  en=off  XmcBlockStatus=1  maskContainerNames=tabcontainer1  block_type=register  block_config=sysgen:Register_config
  DelayB : hdlBasic/Register  init=0  rst=off  en=off  XmcBlockStatus=1  maskContainerNames=tabcontainer1  block_type=register  block_config=sysgen:Register_config
  Mult : hdlBasic/Mult  precision=User Defined  arith_type="Signed  (2's comp)"  n_bits=16  bin_pt=0  quantization=Truncate  overflow=Wrap  en=off  latency=1  opt_float=off  fp_mult_usage=No Usage  use_behavioral_HDL=off  opt=Speed  use_embedded=on  optimum_pipeline=off  pipeline=on  use_rpm=on  placement_style=Triangular  XmcBlockStatus=1  maskContainerNames=group1  block_type=mult  block_config=sysgen:Mult_config  block_width=598  block_height=876
  Mux : hdlBasic/Mux  inputs=2  en=off  latency=1  precision=Full  arith_type=Unsigned  n_bits=16  bin_pt=14  quantization=Truncate  overflow=Wrap  XmcBlockStatus=1  maskContainerNames=tabcontainer1  block_type=mux  block_config=sysgen:Mux_config
  OutA : Outport
  ShiftOut : Outport  Port=2
  ResetOut : Outport  Port=3
  OutB : Outport  Port=4
  wires:
  Accumulator/1 -> Mux/2
  Mult/1 -> Accumulator/1
  InB/1 -> DelayB/1, Mult/2
  Select/1 -> Mux/1
  ShiftIn/1 -> Mux/3
  Mux/1 -> ShiftOut/1
  ResetIn/1 -> Delay/1, Accumulator/2
  InA/1 -> Mult/1, DelayA/1
  DelayA/1 -> OutA/1
  DelayB/1 -> OutB/1
  Delay/1 -> ResetOut/1

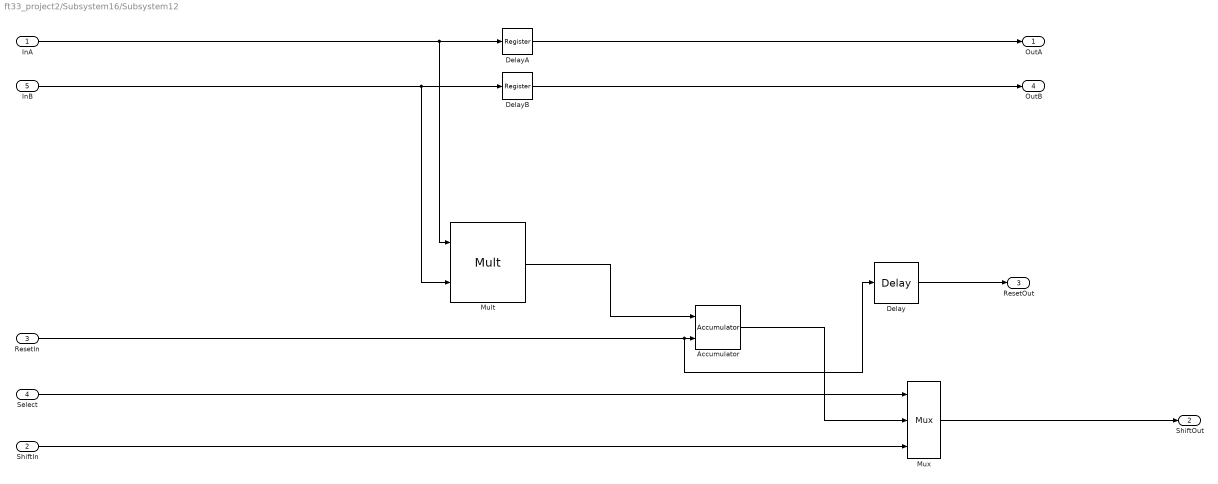
== system ft33_project2/Subsystem16/Subsystem12 ==
  InA : Inport
  ShiftIn : Inport  Port=2
  ResetIn : Inport  Port=3
  Select : Inport  Port=4
  InB : Inport  Port=5
  Accumulator : hdlBasic/Accumulator  operation=Add  n_bits=16  overflow=Wrap  scale=1  rst=on  hasbypass=off  en=off  latency=1  msb_inp=100  msb=100  lsb=-100  use_behavioral_HDL=on  implementation=Fabric  XmcBlockStatus=1  maskContainerNames=group3  block_type=accum  block_config=sysgen:Accum_config  block_width=566  block_height=845
  Delay : hdlBasic/Delay  rst=off  en=off  latency=1  reg_retiming=off  XmcBlockStatus=1  maskContainerNames=group1  block_type=delay  block_config=sysgen:Delay_config
  DelayA : hdlBasic/Register  init=0  rst=off  en=off  XmcBlockStatus=1  maskContainerNames=tabcontainer1  block_type=register  block_config=sysgen:Register_config
  DelayB : hdlBasic/Register  init=0  rst=off  en=off  XmcBlockStatus=1  maskContainerNames=tabcontainer1  block_type=register  block_config=sysgen:Register_config
  Mult : hdlBasic/Mult  precision=User Defined  arith_type="Signed  (2's comp)"  n_bits=16  bin_pt=0  quantization=Truncate  overflow=Wrap  en=off  latency=1  opt_float=off  fp_mult_usage=No Usage  use_behavioral_HDL=off  opt=Speed  use_embedded=on  optimum_pipeline=off  pipeline=on  use_rpm=on  placement_style=Triangular  XmcBlockStatus=1  maskContainerNames=group1  block_type=mult  block_config=sysgen:Mult_config  block_width=598  block_height=876
  Mux : hdlBasic/Mux  inputs=2  en=off  latency=1  precision=Full  arith_type=Unsigned  n_bits=16  bin_pt=14  quantization=Truncate  overflow=Wrap  XmcBlockStatus=1  maskContainerNames=tabcontainer1  block_type=mux  block_config=sysgen:Mux_config
  OutA : Outport
  ShiftOut : Outport  Port=2
  ResetOut : Outport  Port=3
  OutB : Outport  Port=4
  wires:
  Accumulator/1 -> Mux/2
  Mult/1 -> Accumulator/1
  InB/1 -> DelayB/1, Mult/2
  Select/1 -> Mux/1
  ShiftIn/1 -> Mux/3
  Mux/1 -> ShiftOut/1
  ResetIn/1 -> Delay/1, Accumulator/2
  InA/1 -> Mult/1, DelayA/1
  DelayA/1 -> OutA/1
  DelayB/1 -> OutB/1
  Delay/1 -> ResetOut/1

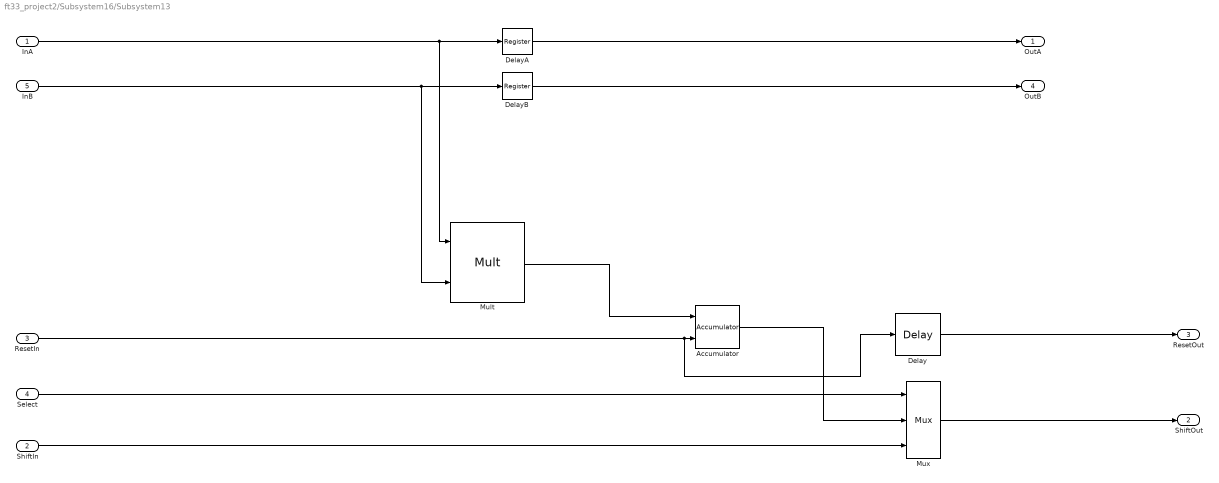
== system ft33_project2/Subsystem16/Subsystem13 ==
  InA : Inport
  ShiftIn : Inport  Port=2
  ResetIn : Inport  Port=3
  Select : Inport  Port=4
  InB : Inport  Port=5
  Accumulator : hdlBasic/Accumulator  operation=Add  n_bits=16  overflow=Flag as error  scale=1  rst=on  hasbypass=off  en=off  latency=1  msb_inp=100  msb=100  lsb=-100  use_behavioral_HDL=on  implementation=Fabric  XmcBlockStatus=1  maskContainerNames=group3  block_type=accum  block_config=sysgen:Accum_config  block_width=566  block_height=845
  Delay : hdlBasic/Delay  rst=off  en=off  latency=1  reg_retiming=off  XmcBlockStatus=1  maskContainerNames=group1  block_type=delay  block_config=sysgen:Delay_config
  DelayA : hdlBasic/Register  init=0  rst=off  en=off  XmcBlockStatus=1  maskContainerNames=tabcontainer1  block_type=register  block_config=sysgen:Register_config
  DelayB : hdlBasic/Register  init=0  rst=off  en=off  XmcBlockStatus=1  maskContainerNames=tabcontainer1  block_type=register  block_config=sysgen:Register_config
  Mult : hdlBasic/Mult  precision=User Defined  arith_type="Signed  (2's comp)"  n_bits=16  bin_pt=0  quantization=Truncate  overflow=Wrap  en=off  latency=1  opt_float=off  fp_mult_usage=No Usage  use_behavioral_HDL=off  opt=Speed  use_embedded=on  optimum_pipeline=off  pipeline=on  use_rpm=on  placement_style=Triangular  XmcBlockStatus=1  maskContainerNames=group1  block_type=mult  block_config=sysgen:Mult_config  block_width=598  block_height=876
  Mux : hdlBasic/Mux  inputs=2  en=off  latency=1  precision=Full  arith_type=Unsigned  n_bits=16  bin_pt=14  quantization=Truncate  overflow=Wrap  XmcBlockStatus=1  maskContainerNames=tabcontainer1  block_type=mux  block_config=sysgen:Mux_config
  OutA : Outport
  ShiftOut : Outport  Port=2
  ResetOut : Outport  Port=3
  OutB : Outport  Port=4
  wires:
  Accumulator/1 -> Mux/2
  Mult/1 -> Accumulator/1
  InB/1 -> DelayB/1, Mult/2
  Select/1 -> Mux/1
  ShiftIn/1 -> Mux/3
  Mux/1 -> ShiftOut/1
  ResetIn/1 -> Delay/1, Accumulator/2
  InA/1 -> Mult/1, DelayA/1
  DelayA/1 -> OutA/1
  DelayB/1 -> OutB/1
  Delay/1 -> ResetOut/1

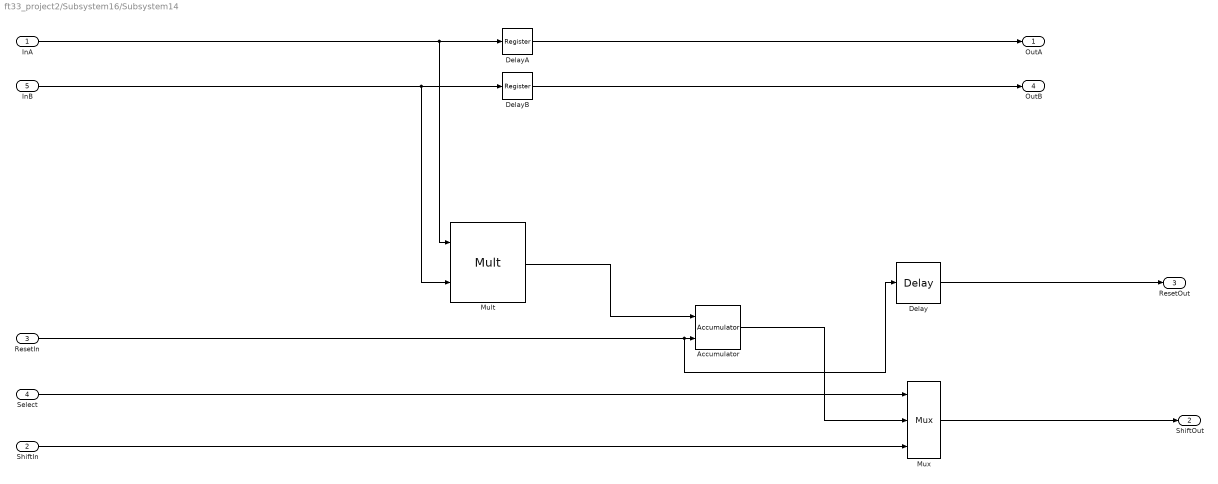
== system ft33_project2/Subsystem16/Subsystem14 ==
  InA : Inport
  ShiftIn : Inport  Port=2
  ResetIn : Inport  Port=3
  Select : Inport  Port=4
  InB : Inport  Port=5
  Accumulator : hdlBasic/Accumulator  operation=Add  n_bits=16  overflow=Wrap  scale=1  rst=on  hasbypass=off  en=off  latency=1  msb_inp=100  msb=100  lsb=-100  use_behavioral_HDL=on  implementation=Fabric  XmcBlockStatus=1  maskContainerNames=group3  block_type=accum  block_config=sysgen:Accum_config  block_width=566  block_height=845
  Delay : hdlBasic/Delay  rst=off  en=off  latency=1  reg_retiming=off  XmcBlockStatus=1  maskContainerNames=group1  block_type=delay  block_config=sysgen:Delay_config
  DelayA : hdlBasic/Register  init=0  rst=off  en=off  XmcBlockStatus=1  maskContainerNames=tabcontainer1  block_type=register  block_config=sysgen:Register_config
  DelayB : hdlBasic/Register  init=0  rst=off  en=off  XmcBlockStatus=1  maskContainerNames=tabcontainer1  block_type=register  block_config=sysgen:Register_config
  Mult : hdlBasic/Mult  precision=User Defined  arith_type="Signed  (2's comp)"  n_bits=16  bin_pt=0  quantization=Truncate  overflow=Wrap  en=off  latency=1  opt_float=off  fp_mult_usage=No Usage  use_behavioral_HDL=off  opt=Speed  use_embedded=on  optimum_pipeline=off  pipeline=on  use_rpm=on  placement_style=Triangular  XmcBlockStatus=1  maskContainerNames=group1  block_type=mult  block_config=sysgen:Mult_config  block_width=598  block_height=876
  Mux : hdlBasic/Mux  inputs=2  en=off  latency=1  precision=Full  arith_type=Unsigned  n_bits=16  bin_pt=14  quantization=Truncate  overflow=Wrap  XmcBlockStatus=1  maskContainerNames=tabcontainer1  block_type=mux  block_config=sysgen:Mux_config
  OutA : Outport
  ShiftOut : Outport  Port=2
  ResetOut : Outport  Port=3
  OutB : Outport  Port=4
  wires:
  Accumulator/1 -> Mux/2
  Mult/1 -> Accumulator/1
  InB/1 -> DelayB/1, Mult/2
  Select/1 -> Mux/1
  ShiftIn/1 -> Mux/3
  Mux/1 -> ShiftOut/1
  ResetIn/1 -> Delay/1, Accumulator/2
  InA/1 -> Mult/1, DelayA/1
  DelayA/1 -> OutA/1
  DelayB/1 -> OutB/1
  Delay/1 -> ResetOut/1

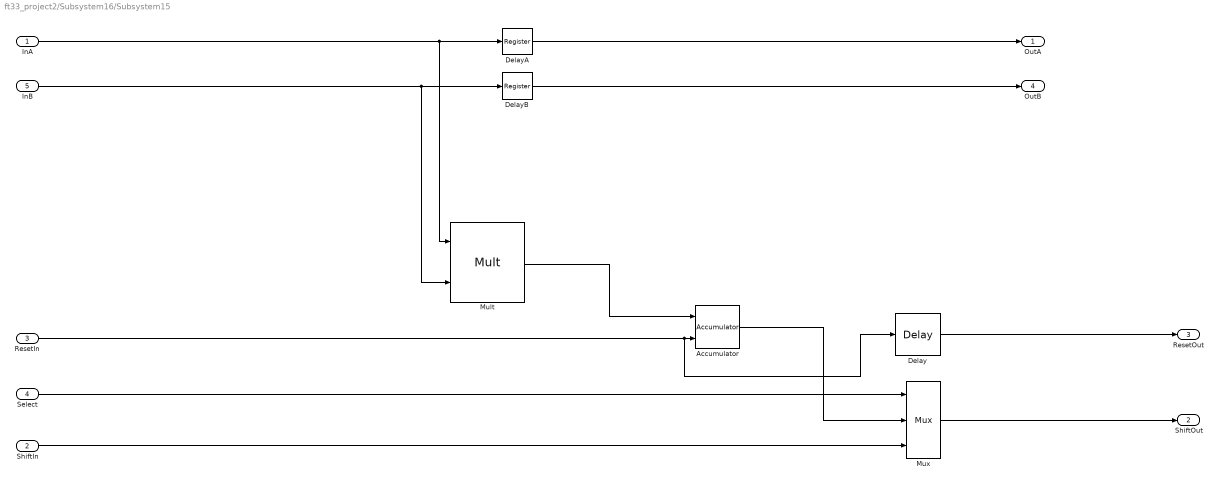
== system ft33_project2/Subsystem16/Subsystem15 ==
  InA : Inport
  ShiftIn : Inport  Port=2
  ResetIn : Inport  Port=3
  Select : Inport  Port=4
  InB : Inport  Port=5
  Accumulator : hdlBasic/Accumulator  operation=Add  n_bits=16  overflow=Flag as error  scale=1  rst=on  hasbypass=off  en=off  latency=1  msb_inp=100  msb=100  lsb=-100  use_behavioral_HDL=on  implementation=Fabric  XmcBlockStatus=1  maskContainerNames=group3  block_type=accum  block_config=sysgen:Accum_config  block_width=566  block_height=845
  Delay : hdlBasic/Delay  rst=off  en=off  latency=1  reg_retiming=off  XmcBlockStatus=1  maskContainerNames=group1  block_type=delay  block_config=sysgen:Delay_config
  DelayA : hdlBasic/Register  init=0  rst=off  en=off  XmcBlockStatus=1  maskContainerNames=tabcontainer1  block_type=register  block_config=sysgen:Register_config
  DelayB : hdlBasic/Register  init=0  rst=off  en=off  XmcBlockStatus=1  maskContainerNames=tabcontainer1  block_type=register  block_config=sysgen:Register_config
  Mult : hdlBasic/Mult  precision=User Defined  arith_type="Signed  (2's comp)"  n_bits=16  bin_pt=0  quantization=Truncate  overflow=Wrap  en=off  latency=1  opt_float=off  fp_mult_usage=No Usage  use_behavioral_HDL=off  opt=Speed  use_embedded=on  optimum_pipeline=off  pipeline=on  use_rpm=on  placement_style=Triangular  XmcBlockStatus=1  maskContainerNames=group1  block_type=mult  block_config=sysgen:Mult_config  block_width=598  block_height=876
  Mux : hdlBasic/Mux  inputs=2  en=off  latency=1  precision=Full  arith_type=Unsigned  n_bits=16  bin_pt=14  quantization=Truncate  overflow=Wrap  XmcBlockStatus=1  maskContainerNames=tabcontainer1  block_type=mux  block_config=sysgen:Mux_config
  OutA : Outport
  ShiftOut : Outport  Port=2
  ResetOut : Outport  Port=3
  OutB : Outport  Port=4
  wires:
  Accumulator/1 -> Mux/2
  Mult/1 -> Accumulator/1
  InB/1 -> DelayB/1, Mult/2
  Select/1 -> Mux/1
  ShiftIn/1 -> Mux/3
  Mux/1 -> ShiftOut/1
  ResetIn/1 -> Delay/1, Accumulator/2
  InA/1 -> Mult/1, DelayA/1
  DelayA/1 -> OutA/1
  DelayB/1 -> OutB/1
  Delay/1 -> ResetOut/1

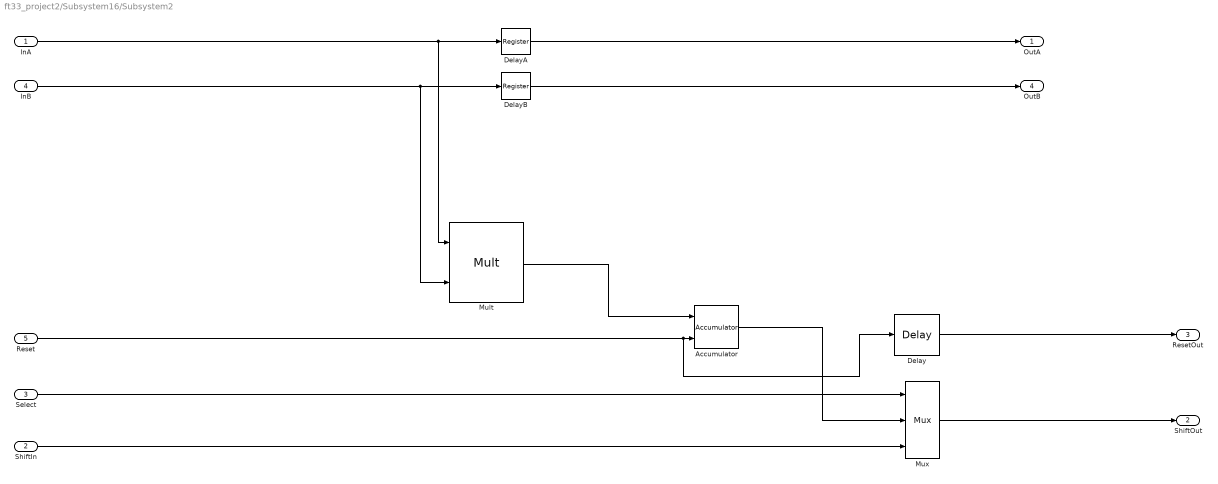
== system ft33_project2/Subsystem16/Subsystem2 ==
  InA : Inport
  ShiftIn : Inport  Port=2
  Select : Inport  Port=3
  InB : Inport  Port=4
  Reset : Inport  Port=5
  Accumulator : hdlBasic/Accumulator  operation=Add  n_bits=16  overflow=Flag as error  scale=1  rst=on  hasbypass=off  en=off  latency=1  msb_inp=100  msb=100  lsb=-100  use_behavioral_HDL=on  implementation=Fabric  XmcBlockStatus=1  maskContainerNames=group3  block_type=accum  block_config=sysgen:Accum_config  block_width=566  block_height=845
  Delay : hdlBasic/Delay  rst=off  en=off  latency=1  reg_retiming=off  XmcBlockStatus=1  maskContainerNames=group1  block_type=delay  block_config=sysgen:Delay_config
  DelayA : hdlBasic/Register  init=0  rst=off  en=off  XmcBlockStatus=1  maskContainerNames=tabcontainer1  block_type=register  block_config=sysgen:Register_config
  DelayB : hdlBasic/Register  init=0  rst=off  en=off  XmcBlockStatus=1  maskContainerNames=tabcontainer1  block_type=register  block_config=sysgen:Register_config
  Mult : hdlBasic/Mult  precision=User Defined  arith_type="Signed  (2's comp)"  n_bits=16  bin_pt=0  quantization=Truncate  overflow=Wrap  en=off  latency=1  opt_float=off  fp_mult_usage=No Usage  use_behavioral_HDL=off  opt=Speed  use_embedded=on  optimum_pipeline=off  pipeline=on  use_rpm=on  placement_style=Triangular  XmcBlockStatus=1  maskContainerNames=group1  block_type=mult  block_config=sysgen:Mult_config  block_width=598  block_height=876
  Mux : hdlBasic/Mux  inputs=2  en=off  latency=1  precision=Full  arith_type=Unsigned  n_bits=16  bin_pt=14  quantization=Truncate  overflow=Wrap  XmcBlockStatus=1  maskContainerNames=tabcontainer1  block_type=mux  block_config=sysgen:Mux_config
  OutA : Outport
  ShiftOut : Outport  Port=2
  ResetOut : Outport  Port=3
  OutB : Outport  Port=4
  wires:
  Accumulator/1 -> Mux/2
  Mult/1 -> Accumulator/1
  InB/1 -> DelayB/1, Mult/2
  Select/1 -> Mux/1
  ShiftIn/1 -> Mux/3
  Mux/1 -> ShiftOut/1
  Reset/1 -> Delay/1, Accumulator/2
  InA/1 -> Mult/1, DelayA/1
  DelayA/1 -> OutA/1
  DelayB/1 -> OutB/1
  Delay/1 -> ResetOut/1

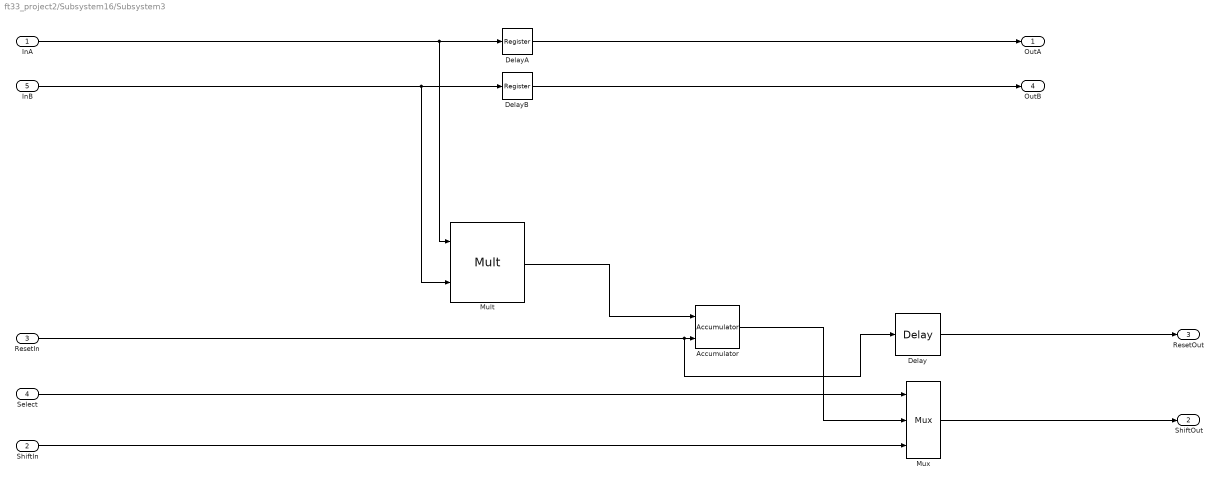
== system ft33_project2/Subsystem16/Subsystem3 ==
  InA : Inport
  ShiftIn : Inport  Port=2
  ResetIn : Inport  Port=3
  Select : Inport  Port=4
  InB : Inport  Port=5
  Accumulator : hdlBasic/Accumulator  operation=Add  n_bits=16  overflow=Flag as error  scale=1  rst=on  hasbypass=off  en=off  latency=1  msb_inp=100  msb=100  lsb=-100  use_behavioral_HDL=on  implementation=Fabric  XmcBlockStatus=1  maskContainerNames=group3  block_type=accum  block_config=sysgen:Accum_config  block_width=566  block_height=845
  Delay : hdlBasic/Delay  rst=off  en=off  latency=1  reg_retiming=off  XmcBlockStatus=1  maskContainerNames=group1  block_type=delay  block_config=sysgen:Delay_config
  DelayA : hdlBasic/Register  init=0  rst=off  en=off  XmcBlockStatus=1  maskContainerNames=tabcontainer1  block_type=register  block_config=sysgen:Register_config
  DelayB : hdlBasic/Register  init=0  rst=off  en=off  XmcBlockStatus=1  maskContainerNames=tabcontainer1  block_type=register  block_config=sysgen:Register_config
  Mult : hdlBasic/Mult  precision=User Defined  arith_type="Signed  (2's comp)"  n_bits=16  bin_pt=0  quantization=Truncate  overflow=Wrap  en=off  latency=1  opt_float=off  fp_mult_usage=No Usage  use_behavioral_HDL=off  opt=Speed  use_embedded=on  optimum_pipeline=off  pipeline=on  use_rpm=on  placement_style=Triangular  XmcBlockStatus=1  maskContainerNames=group1  block_type=mult  block_config=sysgen:Mult_config  block_width=598  block_height=876
  Mux : hdlBasic/Mux  inputs=2  en=off  latency=1  precision=Full  arith_type=Unsigned  n_bits=16  bin_pt=14  quantization=Truncate  overflow=Wrap  XmcBlockStatus=1  maskContainerNames=tabcontainer1  block_type=mux  block_config=sysgen:Mux_config
  OutA : Outport
  ShiftOut : Outport  Port=2
  ResetOut : Outport  Port=3
  OutB : Outport  Port=4
  wires:
  Accumulator/1 -> Mux/2
  Mult/1 -> Accumulator/1
  InB/1 -> DelayB/1, Mult/2
  Select/1 -> Mux/1
  ShiftIn/1 -> Mux/3
  Mux/1 -> ShiftOut/1
  ResetIn/1 -> Delay/1, Accumulator/2
  InA/1 -> Mult/1, DelayA/1
  DelayA/1 -> OutA/1
  DelayB/1 -> OutB/1
  Delay/1 -> ResetOut/1
